simulink model "NetworkModelSimpleIntersection"  (R2018b)
settings: Solver=VariableStepAuto  StartTime=tStart  StopTime=tFinal  FixedStep=0.001  RelTol=1e-3
values from neighbouring files (symbols this model uses):
  Ax = [0 1  0   0 ... (first row only)    [DroneSubsystemModelling.m]
  Ay = [0 1  0   0 ... (first row only)    [DroneSubsystemModelling.m]
  Bx = [0;0;0;b1]    [DroneSubsystemModelling.m]
  By = [0;0;0;b2]    [DroneSubsystemModelling.m]
  ConflictDrone1andDrone2 = ControlDetectionFunction(tout,PositionXDrone1TEST, PositionYDrone1TEST, PositionXDrone2TEST, PositionYDrone2TEST, ConflictDrone1andDrone2)    [ConflictDetectionTEST.m]
  ConflictDrone1andDrone3 = ControlDetectionFunction(tout,PositionXDrone1TEST, PositionYDrone1TEST, PositionXDrone3TEST, PositionYDrone3TEST, ConflictDrone1andDrone3)    [ConflictDetectionTEST.m]
  ConflictDrone1andDrone4 = ControlDetectionFunction(tout,PositionXDrone1TEST, PositionYDrone1TEST, PositionXDrone4TEST, PositionYDrone4TEST, ConflictDrone1andDrone4)    [ConflictDetectionTEST.m]
  ConflictDrone2andDrone3 = ControlDetectionFunction(tout,PositionXDrone2TEST, PositionYDrone2TEST, PositionXDrone3TEST, PositionYDrone3TEST, ConflictDrone2andDrone3)    [ConflictDetectionTEST.m]
  ConflictDrone2andDrone4 = ControlDetectionFunction(tout,PositionXDrone2, PositionYDrone2, PositionXDrone4, PositionYDrone4, ConflictDrone2andDrone4)    [ConflictDetection.m]    (also in ConflictDetectionTEST.m = ControlDetectionFunction(tout,PositionXDrone2TEST, PositionY)
  ConflictDrone3andDrone4 = ControlDetectionFunction(tout,PositionXDrone3TEST, PositionYDrone3TEST, PositionXDrone4TEST, PositionYDrone4TEST, ConflictDrone3andDrone4)    [ConflictDetectionTEST.m]
  Cpx = [1 0 0 0]    [DroneSubsystemModelling.m]
  Cpy = [1 0 0 0]    [DroneSubsystemModelling.m]
  Cvx = [0 1 0 0]    [DroneSubsystemModelling.m]
  Cvy = [0 1 0 0]    [DroneSubsystemModelling.m]
  deltaVx1 = 0.1*cosd (theta2)    [MotionModelling.m]
  deltaVx2 = 0.12*cosd (theta2)    [MotionModelling.m]
  deltaVx3 = 0    [MotionModelling.m]
  deltaVx4 = -0.01*cosd (theta4)    [MotionModelling.m]
  deltaVy1 = 0    [MotionModelling.m]
  deltaVy2 = 0.12*sind (theta2)    [MotionModelling.m]
  deltaVy3 = 0.03*sind (theta3)    [MotionModelling.m]
  deltaVy4 = -0.01*sind (theta4)    [MotionModelling.m]
  VelocityStarX1 = vx10    [MotionModelling.m]
  VelocityStarX2 = vx20    [MotionModelling.m]
  VelocityStarX3 = vx30    [MotionModelling.m]
  VelocityStarX4 = vx40    [MotionModelling.m]
  VelocityStarY1 = vy10    [MotionModelling.m]
  VelocityStarY2 = vy20    [MotionModelling.m]
  VelocityStarY3 = vy30    [MotionModelling.m]
  VelocityStarY4 = vy40    [MotionModelling.m]
  X10 = [x10 vx10 0 0]'    [MotionModelling.m]
  X20 = [x20 vx20 0 0]'    [MotionModelling.m]
  X30 = [x30 vx30 0 0]'    [MotionModelling.m]
  X40 = [x40 vx40 0 0]'    [MotionModelling.m]
  Y10 = [y10 vy10 0 0]'    [MotionModelling.m]
  Y20 = [y20 vy20 0 0]'    [MotionModelling.m]
  Y30 = [y30 vy30 0 0]'    [MotionModelling.m]
  Y40 = [y40 vy40 0 0]'    [MotionModelling.m]
libraries: simulink x8
settings Model: Creator=CowUser  LastModifiedBy=CowUser

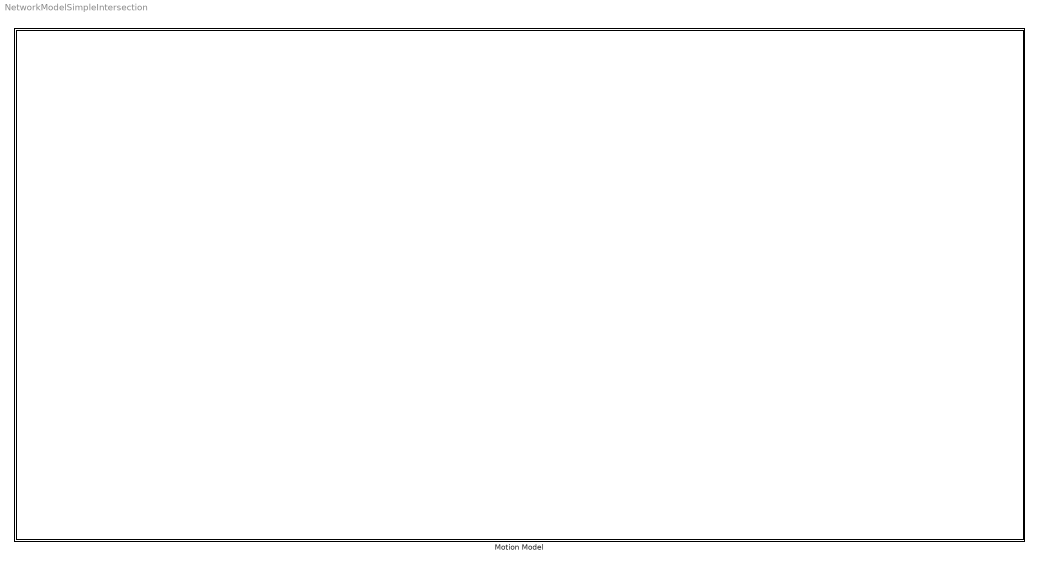
== system NetworkModelSimpleIntersection ==
  Motion Model : Subsystem

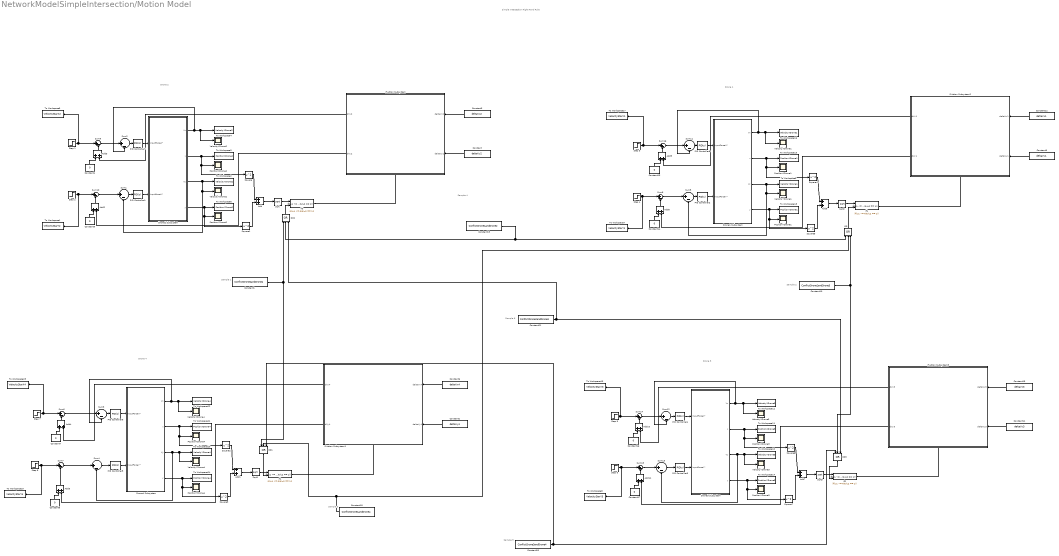
== system NetworkModelSimpleIntersection/Motion Model ==
  note: Drone 2
  note: Simple Intersection
      |
      | Right Hand Rule
  note: Drone 4
  note: Sample 1
  note: Drone 1
  note: Drone 3
  note: Sample 2
  note: Sample 3
  note: Sample 4
  note: Sample 5
  note: Sample 6
  Add{,1..11} (12 alike) : Sum
  Constant : Constant  Value=deltaVy2
  Constant1 : Constant  Value=ConflictDrone2andDrone4
  Constant10 : Constant  Value=ConflictDrone1andDrone3
  Constant11 : Constant  Value=deltaVy3
  Constant12 : Constant  Value=deltaVx1
  Constant{4..5,7..8,13..14,16..17} (8 alike) : Constant  Value=0
  Constant15 : Constant  Value=deltaVx3
  Constant18 : Constant  Value=ConflictDrone1andDrone4
  Constant19 : Constant  Value=ConflictDrone1andDrone2
  Constant2 : Constant  Value=deltaVy4
  Constant20 : Constant  Value=ConflictDrone3andDrone4
  Constant21 : Constant  Value=ConflictDrone2andDrone3
  Constant3 : Constant  Value=deltaVx2
  Constant6 : Constant  Value=deltaVx4
  Constant9 : Constant  Value=deltaVy1
  "Drone1 Subsystem " : Subsystem
  "Drone2 Subsystem " : Subsystem
  Drone3 Subsystem : Subsystem
  "Drone4 Subsystem " : Subsystem
  If Action Subsystem : Subsystem  TreatAsAtomicUnit=on
  If Action Subsystem1 : Subsystem  TreatAsAtomicUnit=on
  If Action Subsystem2 : Subsystem  TreatAsAtomicUnit=on
  If Action Subsystem3 : Subsystem  TreatAsAtomicUnit=on
  If{1..4} (4 alike) : If  NumInputs=2  IfExpression=(u1 <= R)&(u2 == 1)  ShowElse=off
  OR{,1..3} (4 alike) : Logic  Operator=OR  Inputs=3  IconShape=distinctive  AllPortsSameDT=off  OutDataTypeStr='double'
  PID Controller{1..8} (8 alike) : simulink/Continuous/PID Controller  Controller=PID  Form=Parallel  TimeDomain=Continuous-time  SampleTime=-1  IntegratorMethod=Forward Euler  FilterMethod=Forward Euler  ControllerParametersSource=internal  P=1.97139727738968e-05  I=1.5233344900537e-08  D=0.00566857635684116  UseFilter=on  N=15.1370363747334  TunerSelectOption=Transfer Function Based (PID Tuner App)  InitialConditionSource=internal  InitialConditionForIntegrator=0  InitialConditionForFilter=0  DifferentiatorICPrevScaledInput=0  ExternalReset=none  TrackingMode=off  Kt=1  LimitOutput=off  UpperSaturationLimit=inf  LowerSaturationLimit=-inf  LinearizeAsGain=on  AntiWindupMode=none  Kb=1  POutMin=[]  POutMax=[]  IOutMin=[]  IOutMax=[]  DOutMin=[]  DOutMax=[]  NOutMin=[]  NOutMax=[]  SumOutMin=[]  SumOutMax=[]  SaturationOutMin=[]  SaturationOutMax=[]  PParamMin=[]  PParamMax=[]  IParamMin=[]  IParamMax=[]  DParamMin=[]  DParamMax=[]  NParamMin=[]  NParamMax=[]  KbParamMin=[]  KbParamMax=[]  KtParamMin=[]  KtParamMax=[]  KbOutMin=[]  KbOutMax=[]  KtOutMin=[]  KtOutMax=[]  IntegratorOutMin=[]  IntegratorOutMax=[]  FilterOutMin=[]  FilterOutMax=[]  SumI1OutMin=[]  SumI1OutMax=[]  SumI2OutMin=[]  SumI2OutMax=[]  SumI3OutMin=[]  SumI3OutMax=[]  SumI4OutMin=[]  SumI4OutMax=[]  SumDOutMin=[]  SumDOutMax=[]  DifferentiatorOutMin=[]  DifferentiatorOutMax=[]  FilterDiffOutCoefMin=[]  FilterDiffOutCoefMax=[]  ReciprocalOutMin=[]  ReciprocalOutMax=[]  SumDenOutMin=[]  SumDenOutMax=[]  SumNumOutMin=[]  SumNumOutMax=[]  DivideOutMin=[]  DivideOutMax=[]  IntegratorContinuousStateAttributes=''  IntegratorStateMustResolveToSignalObject=off  IntegratorRTWStateStorageClass=Auto  FilterContinuousStateAttributes=''  FilterStateMustResolveToSignalObject=off  FilterRTWStateStorageClass=Auto  ParallelPVariant=InternalParameters  IdealPVariant=Disabled  IVariant=InternalParameters  DVariant=InternalParameters  IntegratorVariant=Continuous  SatVariant=Disabled  AWVariant=Passthrough  PCopyVariant=Disabled  TRVariant=Disabled  FdbkBlocksVariant=Forward  IdealPFdbkVariant=Disabled  SatFdbkVariant=Disabled  DerivativeFilterVariant=ContFilter  NVariant=InternalParameters  NCopyVariant=Disabled  FilterICVariant=InternalICsFilter  IntegratorICVariant=InternalICs  ExternalResetVariant=Disabled  TRSumVariant=Passthrough  SumFdbkVariant=Disabled  SumVariant=Sum_PID
  PositionXDrone{1..4} (4 alike) : Scope
  PositionYDrone{1..4} (4 alike) : Scope
  Sqrt{,1..3} (4 alike) : Sqrt  SaturateOnIntegerOverflow=on
  Square{,1..7} (8 alike) : Math  Operator=square  SaturateOnIntegerOverflow=on
  Step 1 : Step  Time=0  After=VelocityStarX2  SampleTime=0
  Step 2 : Step  Time=0  After=VelocityStarY2  SampleTime=0
  Step 3 : Step  Time=0  After=VelocityStarX1  SampleTime=0
  Step 4 : Step  Time=0  After=VelocityStarY1  SampleTime=0
  Step 5 : Step  Time=0  After=VelocityStarX3  SampleTime=0
  Step 6 : Step  Time=0  After=VelocityStarY3  SampleTime=0
  Step 7 : Step  Time=0  After=VelocityStarX4  SampleTime=0
  Step 8 : Step  Time=0  After=VelocityStarY4  SampleTime=0
  Sum{1..16} (16 alike) : Sum  Inputs=|+-
  To Workspace1 : ToWorkspace  VariableName=VelocityStarY2  SampleTime=-1
  To Workspace10 : ToWorkspace  VariableName=VelocityYDrone3  SampleTime=-1
  To Workspace11 : ToWorkspace  VariableName=PositionXDrone3  SampleTime=-1
  To Workspace12 : ToWorkspace  VariableName=VelocityXDrone3  SampleTime=-1
  To Workspace13 : ToWorkspace  VariableName=VelocityStarX3  SampleTime=-1
  To Workspace14 : ToWorkspace  VariableName=PositionYDrone3  SampleTime=-1
  To Workspace15 : ToWorkspace  VariableName=PositionXDrone1  SampleTime=-1
  To Workspace16 : ToWorkspace  VariableName=VelocityXDrone1  SampleTime=-1
  To Workspace17 : ToWorkspace  VariableName=VelocityStarX1  SampleTime=-1
  To Workspace18 : ToWorkspace  VariableName=PositionYDrone1  SampleTime=-1
  To Workspace19 : ToWorkspace  VariableName=VelocityStarY4  SampleTime=-1
  To Workspace2 : ToWorkspace  VariableName=VelocityYDrone2  SampleTime=-1
  To Workspace20 : ToWorkspace  VariableName=VelocityYDrone4  SampleTime=-1
  To Workspace21 : ToWorkspace  VariableName=PositionXDrone4  SampleTime=-1
  To Workspace22 : ToWorkspace  VariableName=VelocityXDrone4  SampleTime=-1
  To Workspace23 : ToWorkspace  VariableName=VelocityStarX4  SampleTime=-1
  To Workspace24 : ToWorkspace  VariableName=PositionYDrone4  SampleTime=-1
  To Workspace3 : ToWorkspace  VariableName=PositionXDrone2  SampleTime=-1
  To Workspace4 : ToWorkspace  VariableName=VelocityXDrone2  SampleTime=-1
  To Workspace5 : ToWorkspace  VariableName=VelocityStarX2  SampleTime=-1
  To Workspace6 : ToWorkspace  VariableName=PositionYDrone2  SampleTime=-1
  To Workspace7 : ToWorkspace  VariableName=VelocityStarY1  SampleTime=-1
  To Workspace8 : ToWorkspace  VariableName=VelocityStarY3  SampleTime=-1
  To Workspace9 : ToWorkspace  VariableName=VelocityYDrone1  SampleTime=-1
  VelocityXDrone{1..4} (4 alike) : Scope
  VelocityYDrone{1..4} (4 alike) : Scope
  wires:
  "Drone2 Subsystem "/3(Vy) -> Sum1/2, VelocityYDrone2/1, To Workspace2/1
  Sum1/1 -> PID Controller1/1
  PID Controller7/1 -> "Drone2 Subsystem "/1(InputForceX*)
  "Drone2 Subsystem "/4(y) -> Square1/1, PositionYDrone2/1, To Workspace6/1
  "Drone2 Subsystem "/2(x) -> Square/1, PositionXDrone2/1, To Workspace3/1
  PID Controller1/1 -> "Drone2 Subsystem "/2("InputForceY* ")
  "Drone2 Subsystem "/1(Vx) -> VelocityXDrone2/1, To Workspace4/1, Sum2/2
  Step 7/1 -> Sum6/1, To Workspace23/1
  Step 8/1 -> To Workspace19/1, Sum7/1
  Square/1 -> Add/1
  Square1/1 -> Add/2
  Add/1 -> Sqrt/1
  Sqrt/1 -> If3/1
  Square2/1 -> Add1/1
  Add1/1 -> Sqrt1/1
  "Drone4 Subsystem "/2(x) -> Square2/1, PositionXDrone4/1, To Workspace21/1
  Square3/1 -> Add1/2
  "Drone4 Subsystem "/4(y) -> Square3/1, PositionYDrone4/1, To Workspace24/1
  Sqrt1/1 -> If1/1
  Sum2/1 -> PID Controller7/1
  Constant/1 -> If Action Subsystem/2(deltaVy2)
  Constant3/1 -> If Action Subsystem/1(deltaVx2)
  Step 1/1 -> Sum9/1, To Workspace5/1
  Sum10/1 -> Sum1/1
  Step 2/1 -> Sum10/1, To Workspace1/1
  If Action Subsystem/1(dVx2) -> Add3/2
  If Action Subsystem/2(dVy2) -> Add2/2
  If3/1 -> If Action Subsystem/Action
  Constant4/1 -> Add3/1
  Constant5/1 -> Add2/1
  Add2/1 -> Sum10/2
  Constant1/1 -> OR1/1, OR2/1
  If1/1 -> If Action Subsystem1/Action
  If Action Subsystem1/1(dVx4) -> Add4/2
  Constant2/1 -> If Action Subsystem1/2(deltaVy4)
  Constant6/1 -> If Action Subsystem1/1(deltaVx4)
  Add4/1 -> Sum6/2
  Constant7/1 -> Add4/1
  Sum3/1 -> PID Controller6/1
  "Drone4 Subsystem "/1(Vx) -> Sum3/2, To Workspace22/1, VelocityXDrone4/1
  Constant8/1 -> Add5/1
  If Action Subsystem1/2(dVy4) -> Add5/2
  "Drone4 Subsystem "/3(Vy) -> Sum4/2, VelocityYDrone4/1, To Workspace20/1
  Sum4/1 -> PID Controller3/1
  Add3/1 -> Sum9/2
  Sum9/1 -> Sum2/1
  Step 3/1 -> Sum16/1, To Workspace17/1
  Add9/1 -> Sum16/2
  "Drone1 Subsystem "/4(y) -> Square5/1, PositionYDrone1/1, To Workspace18/1
  Drone3 Subsystem/3(Vy) -> Sum13/2, VelocityYDrone3/1, To Workspace10/1
  Constant17/1 -> Add11/1
  Add10/1 -> Sum14/2
  Sum15/1 -> Sum13/1
  If Action Subsystem3/2(dVy3) -> Add11/2
  PID Controller8/1 -> "Drone1 Subsystem "/1(InputForceX*)
  Add11/1 -> Sum15/2
  Sum11/1 -> PID Controller8/1
  Constant10/1 -> OR3/2, OR/3
  If Action Subsystem2/1(dVx1) -> Add9/2
  Constant11/1 -> If Action Subsystem3/2(deltaVy3)
  Constant13/1 -> Add9/1
  Sqrt3/1 -> If2/1
  Constant16/1 -> Add10/1
  PID Controller2/1 -> "Drone1 Subsystem "/2("InputForceY* ")
  Add8/1 -> Sum8/2
  Drone3 Subsystem/1(Vx) -> Sum12/2, To Workspace12/1, VelocityXDrone3/1
  Constant14/1 -> Add8/1
  If2/1 -> If Action Subsystem3/Action
  If Action Subsystem3/1(dVx3) -> Add10/2
  Drone3 Subsystem/4(y) -> Square7/1, PositionYDrone3/1, To Workspace14/1
  Constant12/1 -> If Action Subsystem2/1(deltaVx1)
  Constant15/1 -> If Action Subsystem3/1(deltaVx3)
  Step 4/1 -> Sum8/1, To Workspace7/1
  "Drone1 Subsystem "/2(x) -> Square4/1, PositionXDrone1/1, To Workspace15/1
  Add7/1 -> Sqrt3/1
  Square6/1 -> Add7/1
  Square5/1 -> Add6/2
  Constant9/1 -> If Action Subsystem2/2(deltaVy1)
  Square7/1 -> Add7/2
  Sum13/1 -> PID Controller5/1
  Drone3 Subsystem/2(x) -> Square6/1, PositionXDrone3/1, To Workspace11/1
  Sum14/1 -> Sum12/1
  Step 5/1 -> Sum14/1, To Workspace13/1
  Sum12/1 -> PID Controller4/1
  Step 6/1 -> To Workspace8/1, Sum15/1
  Sum5/1 -> PID Controller2/1
  Sqrt2/1 -> If4/1
  PID Controller4/1 -> Drone3 Subsystem/1(InputForceX*)
  Add6/1 -> Sqrt2/1
  PID Controller5/1 -> Drone3 Subsystem/2("InputForceY* ")
  "Drone1 Subsystem "/3(Vy) -> Sum5/2, VelocityYDrone1/1, To Workspace9/1
  If Action Subsystem2/2(dVy1) -> Add8/2
  Square4/1 -> Add6/1
  If4/1 -> If Action Subsystem2/Action
  "Drone1 Subsystem "/1(Vx) -> VelocityXDrone1/1, To Workspace16/1, Sum11/2
  OR/1 -> If4/2
  Constant18/1 -> OR/2, OR1/2
  OR1/1 -> If1/2
  OR2/1 -> If3/2
  Constant19/1 -> OR2/2, OR/1
  Constant20/1 -> OR3/1, OR1/3
  OR3/1 -> If2/2
  Constant21/1 -> OR3/3, OR2/3
  Sum6/1 -> Sum3/1
  Sum8/1 -> Sum5/1
  Sum16/1 -> Sum11/1
  Add5/1 -> Sum7/2
  Sum7/1 -> Sum4/1
  PID Controller6/1 -> "Drone4 Subsystem "/1(InputForceX*)
  PID Controller3/1 -> "Drone4 Subsystem "/2("InputForceY* ")

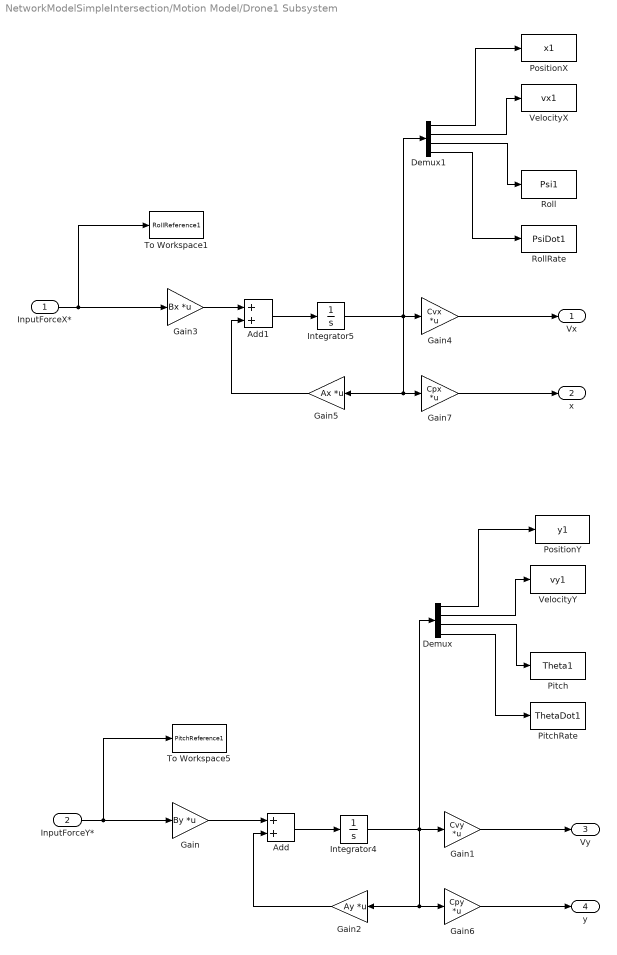
== system NetworkModelSimpleIntersection/Motion Model/Drone1 Subsystem  ==
  InputForceX* : Inport
  "InputForceY* " : Inport  Port=2
  Add : Sum
  Add1 : Sum
  Demux : Demux
  Demux1 : Demux
  Gain : Gain  Gain=By  Multiplication=Matrix(K*u)
  Gain1 : Gain  Gain=Cvy  Multiplication=Matrix(K*u)
  Gain2 : Gain  Gain=Ay  Multiplication=Matrix(K*u)
  Gain3 : Gain  Gain=Bx  Multiplication=Matrix(K*u)
  Gain4 : Gain  Gain=Cvx  Multiplication=Matrix(K*u)
  Gain5 : Gain  Gain=Ax  Multiplication=Matrix(K*u)
  Gain6 : Gain  Gain=Cpy  Multiplication=Matrix(K*u)
  Gain7 : Gain  Gain=Cpx  Multiplication=Matrix(K*u)
  Integrator4 : Integrator  InitialCondition=Y10
  Integrator5 : Integrator  InitialCondition=X10
  Pitch : ToWorkspace  VariableName=Theta1  SampleTime=-1
  PitchRate : ToWorkspace  VariableName=ThetaDot1  SampleTime=-1
  PositionX : ToWorkspace  VariableName=x1  SampleTime=-1
  PositionY : ToWorkspace  VariableName=y1  SampleTime=-1
  Roll : ToWorkspace  VariableName=Psi1  SampleTime=-1
  RollRate : ToWorkspace  VariableName=PsiDot1  SampleTime=-1
  To Workspace1 : ToWorkspace  VariableName=RollReference1  SampleTime=-1
  To Workspace5 : ToWorkspace  VariableName=PitchReference1  SampleTime=-1
  VelocityX : ToWorkspace  VariableName=vx1  SampleTime=-1
  VelocityY : ToWorkspace  VariableName=vy1  SampleTime=-1
  Vx : Outport
  x : Outport  Port=2
  Vy : Outport  Port=3
  y : Outport  Port=4
  wires:
  Gain1/1 -> Vy/1
  Demux1/1 -> PositionX/1
  Demux1/2 -> VelocityX/1
  Gain/1 -> Add/1
  Integrator5/1 -> Gain4/1, Gain5/1, Gain7/1, Demux1/1
  Add/1 -> Integrator4/1
  Demux1/4 -> RollRate/1
  "InputForceY* "/1 -> Gain/1, To Workspace5/1
  Demux/1 -> PositionY/1
  Gain6/1 -> y/1
  Demux/3 -> Pitch/1
  Gain7/1 -> x/1
  Add1/1 -> Integrator5/1
  Integrator4/1 -> Gain6/1, Gain2/1, Demux/1, Gain1/1
  Gain5/1 -> Add1/2
  Gain4/1 -> Vx/1
  InputForceX*/1 -> Gain3/1, To Workspace1/1
  Demux1/3 -> Roll/1
  Demux/4 -> PitchRate/1
  Gain3/1 -> Add1/1
  Gain2/1 -> Add/2
  Demux/2 -> VelocityY/1

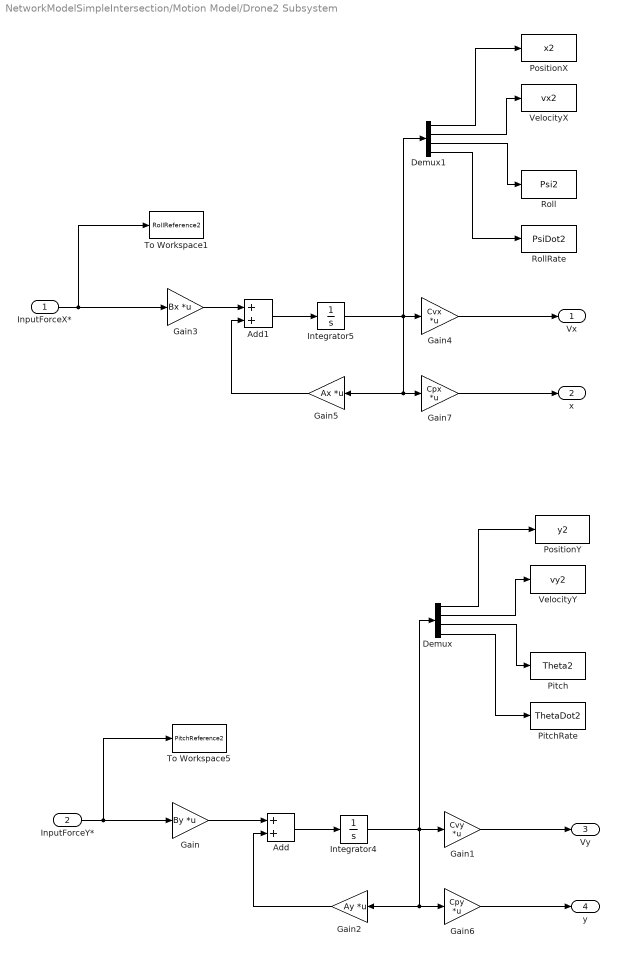
== system NetworkModelSimpleIntersection/Motion Model/Drone2 Subsystem  ==
  InputForceX* : Inport
  "InputForceY* " : Inport  Port=2
  Add : Sum
  Add1 : Sum
  Demux : Demux
  Demux1 : Demux
  Gain : Gain  Gain=By  Multiplication=Matrix(K*u)
  Gain1 : Gain  Gain=Cvy  Multiplication=Matrix(K*u)
  Gain2 : Gain  Gain=Ay  Multiplication=Matrix(K*u)
  Gain3 : Gain  Gain=Bx  Multiplication=Matrix(K*u)
  Gain4 : Gain  Gain=Cvx  Multiplication=Matrix(K*u)
  Gain5 : Gain  Gain=Ax  Multiplication=Matrix(K*u)
  Gain6 : Gain  Gain=Cpy  Multiplication=Matrix(K*u)
  Gain7 : Gain  Gain=Cpx  Multiplication=Matrix(K*u)
  Integrator4 : Integrator  InitialCondition=Y20
  Integrator5 : Integrator  InitialCondition=X20
  Pitch : ToWorkspace  VariableName=Theta2  SampleTime=-1
  PitchRate : ToWorkspace  VariableName=ThetaDot2  SampleTime=-1
  PositionX : ToWorkspace  VariableName=x2  SampleTime=-1
  PositionY : ToWorkspace  VariableName=y2  SampleTime=-1
  Roll : ToWorkspace  VariableName=Psi2  SampleTime=-1
  RollRate : ToWorkspace  VariableName=PsiDot2  SampleTime=-1
  To Workspace1 : ToWorkspace  VariableName=RollReference2  SampleTime=-1
  To Workspace5 : ToWorkspace  VariableName=PitchReference2  SampleTime=-1
  VelocityX : ToWorkspace  VariableName=vx2  SampleTime=-1
  VelocityY : ToWorkspace  VariableName=vy2  SampleTime=-1
  Vx : Outport
  x : Outport  Port=2
  Vy : Outport  Port=3
  y : Outport  Port=4
  wires:
  Demux/1 -> PositionY/1
  Demux1/2 -> VelocityX/1
  Demux1/4 -> RollRate/1
  Demux1/3 -> Roll/1
  Gain4/1 -> Vx/1
  "InputForceY* "/1 -> Gain/1, To Workspace5/1
  Gain/1 -> Add/1
  Demux/4 -> PitchRate/1
  Demux/3 -> Pitch/1
  Add/1 -> Integrator4/1
  Demux1/1 -> PositionX/1
  Gain1/1 -> Vy/1
  InputForceX*/1 -> Gain3/1, To Workspace1/1
  Gain7/1 -> x/1
  Integrator4/1 -> Gain6/1, Gain2/1, Demux/1, Gain1/1
  Demux/2 -> VelocityY/1
  Gain6/1 -> y/1
  Gain3/1 -> Add1/1
  Add1/1 -> Integrator5/1
  Gain2/1 -> Add/2
  Integrator5/1 -> Gain4/1, Gain5/1, Gain7/1, Demux1/1
  Gain5/1 -> Add1/2

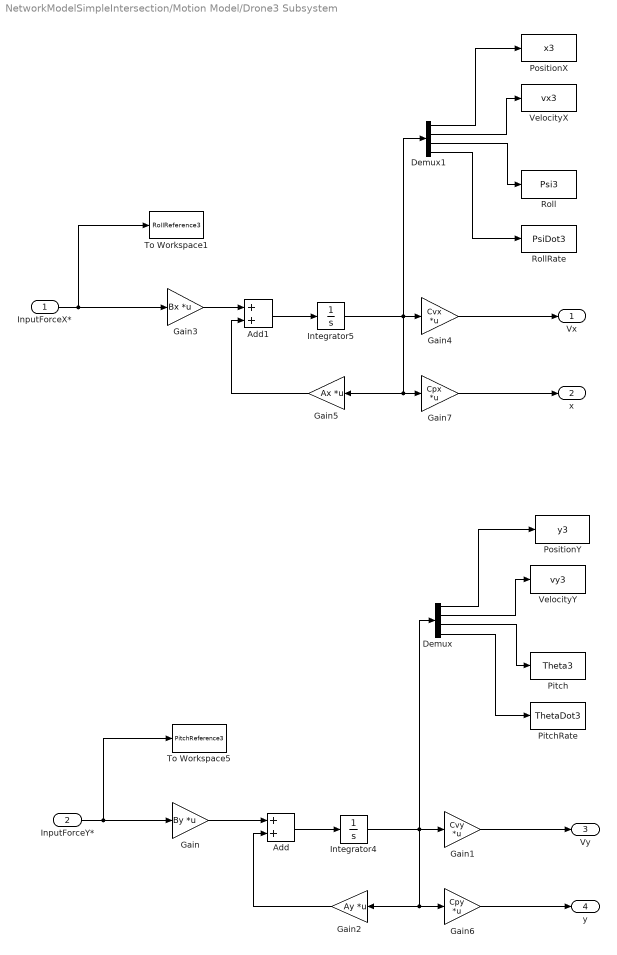
== system NetworkModelSimpleIntersection/Motion Model/Drone3 Subsystem ==
  InputForceX* : Inport
  "InputForceY* " : Inport  Port=2
  Add : Sum
  Add1 : Sum
  Demux : Demux
  Demux1 : Demux
  Gain : Gain  Gain=By  Multiplication=Matrix(K*u)
  Gain1 : Gain  Gain=Cvy  Multiplication=Matrix(K*u)
  Gain2 : Gain  Gain=Ay  Multiplication=Matrix(K*u)
  Gain3 : Gain  Gain=Bx  Multiplication=Matrix(K*u)
  Gain4 : Gain  Gain=Cvx  Multiplication=Matrix(K*u)
  Gain5 : Gain  Gain=Ax  Multiplication=Matrix(K*u)
  Gain6 : Gain  Gain=Cpy  Multiplication=Matrix(K*u)
  Gain7 : Gain  Gain=Cpx  Multiplication=Matrix(K*u)
  Integrator4 : Integrator  InitialCondition=Y30
  Integrator5 : Integrator  InitialCondition=X30
  Pitch : ToWorkspace  VariableName=Theta3  SampleTime=-1
  PitchRate : ToWorkspace  VariableName=ThetaDot3  SampleTime=-1
  PositionX : ToWorkspace  VariableName=x3  SampleTime=-1
  PositionY : ToWorkspace  VariableName=y3  SampleTime=-1
  Roll : ToWorkspace  VariableName=Psi3  SampleTime=-1
  RollRate : ToWorkspace  VariableName=PsiDot3  SampleTime=-1
  To Workspace1 : ToWorkspace  VariableName=RollReference3  SampleTime=-1
  To Workspace5 : ToWorkspace  VariableName=PitchReference3  SampleTime=-1
  VelocityX : ToWorkspace  VariableName=vx3  SampleTime=-1
  VelocityY : ToWorkspace  VariableName=vy3  SampleTime=-1
  Vx : Outport
  x : Outport  Port=2
  Vy : Outport  Port=3
  y : Outport  Port=4
  wires:
  Demux/2 -> VelocityY/1
  Gain2/1 -> Add/2
  Gain6/1 -> y/1
  Gain3/1 -> Add1/1
  Demux/4 -> PitchRate/1
  Add1/1 -> Integrator5/1
  Gain/1 -> Add/1
  Integrator4/1 -> Gain6/1, Gain2/1, Demux/1, Gain1/1
  Demux1/3 -> Roll/1
  InputForceX*/1 -> Gain3/1, To Workspace1/1
  Demux1/1 -> PositionX/1
  Integrator5/1 -> Gain4/1, Gain5/1, Gain7/1, Demux1/1
  Gain5/1 -> Add1/2
  Demux/3 -> Pitch/1
  Gain7/1 -> x/1
  Demux1/2 -> VelocityX/1
  Add/1 -> Integrator4/1
  Gain4/1 -> Vx/1
  "InputForceY* "/1 -> Gain/1, To Workspace5/1
  Demux/1 -> PositionY/1
  Demux1/4 -> RollRate/1
  Gain1/1 -> Vy/1

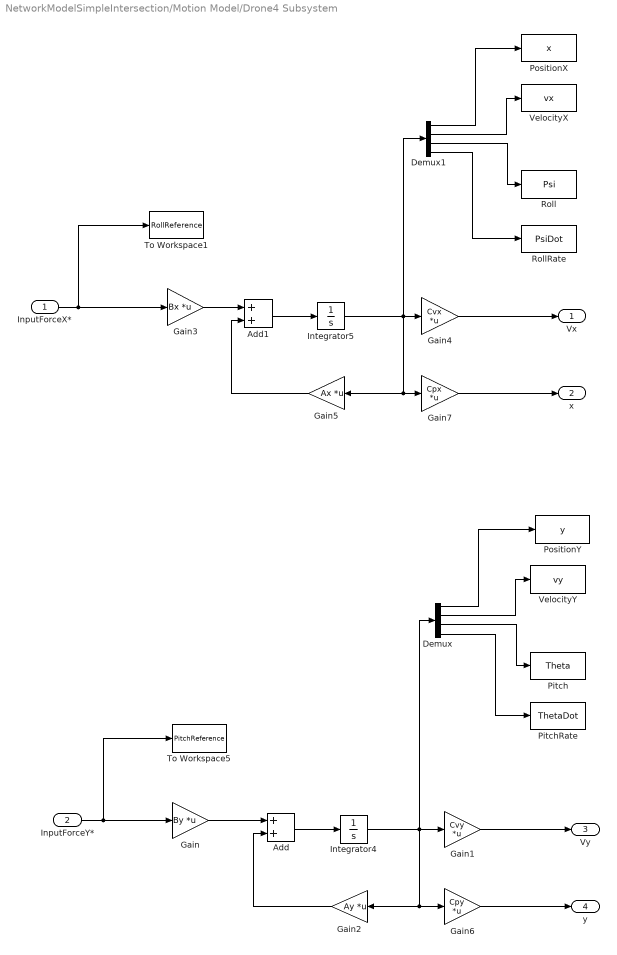
== system NetworkModelSimpleIntersection/Motion Model/Drone4 Subsystem  ==
  InputForceX* : Inport
  "InputForceY* " : Inport  Port=2
  Add : Sum
  Add1 : Sum
  Demux : Demux
  Demux1 : Demux
  Gain : Gain  Gain=By  Multiplication=Matrix(K*u)
  Gain1 : Gain  Gain=Cvy  Multiplication=Matrix(K*u)
  Gain2 : Gain  Gain=Ay  Multiplication=Matrix(K*u)
  Gain3 : Gain  Gain=Bx  Multiplication=Matrix(K*u)
  Gain4 : Gain  Gain=Cvx  Multiplication=Matrix(K*u)
  Gain5 : Gain  Gain=Ax  Multiplication=Matrix(K*u)
  Gain6 : Gain  Gain=Cpy  Multiplication=Matrix(K*u)
  Gain7 : Gain  Gain=Cpx  Multiplication=Matrix(K*u)
  Integrator4 : Integrator  InitialCondition=Y40
  Integrator5 : Integrator  InitialCondition=X40
  Pitch : ToWorkspace  VariableName=Theta  SampleTime=-1
  PitchRate : ToWorkspace  VariableName=ThetaDot  SampleTime=-1
  PositionX : ToWorkspace  VariableName=x  SampleTime=-1
  PositionY : ToWorkspace  VariableName=y  SampleTime=-1
  Roll : ToWorkspace  VariableName=Psi  SampleTime=-1
  RollRate : ToWorkspace  VariableName=PsiDot  SampleTime=-1
  To Workspace1 : ToWorkspace  VariableName=RollReference  SampleTime=-1
  To Workspace5 : ToWorkspace  VariableName=PitchReference  SampleTime=-1
  VelocityX : ToWorkspace  VariableName=vx  SampleTime=-1
  VelocityY : ToWorkspace  VariableName=vy  SampleTime=-1
  Vx : Outport
  x : Outport  Port=2
  Vy : Outport  Port=3
  y : Outport  Port=4
  wires:
  Gain4/1 -> Vx/1
  Demux/2 -> VelocityY/1
  Demux/4 -> PitchRate/1
  Gain3/1 -> Add1/1
  InputForceX*/1 -> Gain3/1, To Workspace1/1
  Gain2/1 -> Add/2
  Demux1/3 -> Roll/1
  Gain7/1 -> x/1
  Add1/1 -> Integrator5/1
  Demux/3 -> Pitch/1
  Gain5/1 -> Add1/2
  Gain6/1 -> y/1
  Integrator5/1 -> Gain4/1, Gain5/1, Gain7/1, Demux1/1
  Gain/1 -> Add/1
  Demux/1 -> PositionY/1
  Add/1 -> Integrator4/1
  Demux1/4 -> RollRate/1
  "InputForceY* "/1 -> Gain/1, To Workspace5/1
  Integrator4/1 -> Gain6/1, Gain2/1, Demux/1, Gain1/1
  Demux1/1 -> PositionX/1
  Demux1/2 -> VelocityX/1
  Gain1/1 -> Vy/1

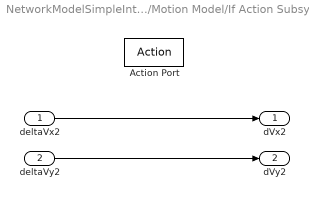
== system NetworkModelSimpleIntersection/Motion Model/If Action Subsystem ==
  deltaVx2 : Inport
  deltaVy2 : Inport  Port=2
  Action Port : ActionPort  ActionType=then
  dVx2 : Outport
  dVy2 : Outport  Port=2
  wires:
  deltaVx2/1 -> dVx2/1
  deltaVy2/1 -> dVy2/1

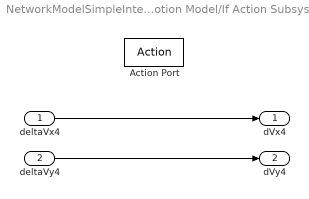
== system NetworkModelSimpleIntersection/Motion Model/If Action Subsystem1 ==
  deltaVx4 : Inport
  deltaVy4 : Inport  Port=2
  Action Port : ActionPort  ActionType=then
  dVx4 : Outport
  dVy4 : Outport  Port=2
  wires:
  deltaVx4/1 -> dVx4/1
  deltaVy4/1 -> dVy4/1

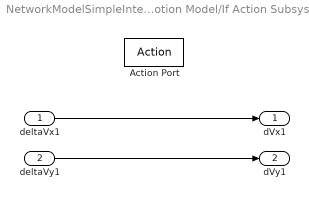
== system NetworkModelSimpleIntersection/Motion Model/If Action Subsystem2 ==
  deltaVx1 : Inport
  deltaVy1 : Inport  Port=2
  Action Port : ActionPort  ActionType=then
  dVx1 : Outport
  dVy1 : Outport  Port=2
  wires:
  deltaVx1/1 -> dVx1/1
  deltaVy1/1 -> dVy1/1

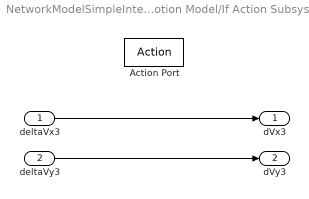
== system NetworkModelSimpleIntersection/Motion Model/If Action Subsystem3 ==
  deltaVx3 : Inport
  deltaVy3 : Inport  Port=2
  Action Port : ActionPort  ActionType=then
  dVx3 : Outport
  dVy3 : Outport  Port=2
  wires:
  deltaVx3/1 -> dVx3/1
  deltaVy3/1 -> dVy3/1
